simulink subsystem "BackwardAccConverter"  (R2025a)
settings: Solver=VariableStepAuto  StartTime=0.0  StopTime=10.0  RelTol=1e-3
model mask{k_rack=0, i_gear=0}
settings Model: Creator=Глеб  LastModifiedBy=Глеб

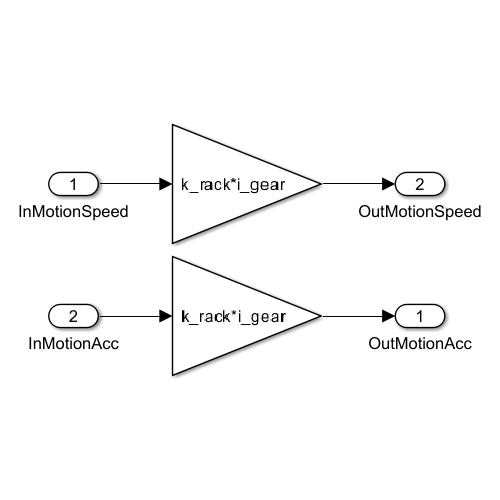
[thumbnail: Simulink's stored preview of the top-level diagram]
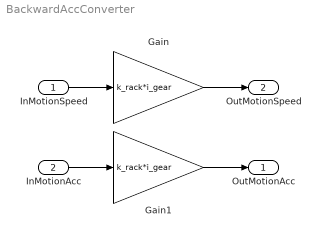
== system BackwardAccConverter ==
  InMotionSpeed : Inport
  InMotionAcc : Inport  Port=2
  Gain : Gain  Gain=k_rack*i_gear
  Gain1 : Gain  Gain=k_rack*i_gear
  OutMotionAcc : Outport
  OutMotionSpeed : Outport  Port=2
  wires:
  InMotionSpeed/1 -> Gain/1
  Gain/1 -> OutMotionSpeed/1
  Gain1/1 -> OutMotionAcc/1
  InMotionAcc/1 -> Gain1/1
